simulink model "Lab5_Q4"  (R2021a)
settings: Solver=VariableStepAuto  StartTime=0.0  StopTime=10.0  RelTol=1e-3
settings Model: Creator=student  LastModifiedBy=student

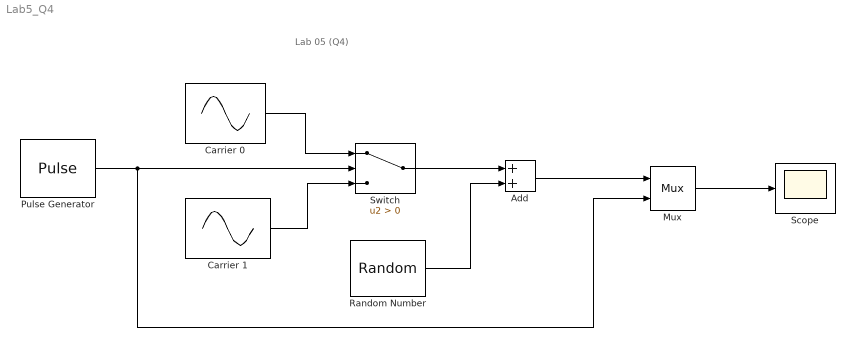
== system Lab5_Q4 ==
  note: Lab 05 (Q4)
  Add : Sum
  Carrier 0 : Sin  Frequency=3131.5926  SampleTime=0.01
  Carrier 1 : Sin  Frequency=9424.7779  SampleTime=0.01
  Mux : Mux  Inputs=2
  Pulse Generator : DiscretePulseGenerator  PulseType=Time based  PulseWidth=50
  Random Number : RandomNumber  Variance=0.1  SampleTime=1e-5
  Scope : Scope
  Switch : Switch  Criteria=u2 > Threshold
  wires:
  Mux/1 -> Scope/1
  Add/1 -> Mux/1
  Pulse Generator/1 -> Mux/2, Switch/2
  Switch/1 -> Add/1
  Carrier 0/1 -> Switch/1
  Random Number/1 -> Add/2
  Carrier 1/1 -> Switch/3
